simulink model "Control_Robot_using_Simulink"  (R2018b)
settings: Solver=FixedStepAuto  StartTime=0.0  StopTime=inf  FixedStep=0.01  RelTol=1e-3
undefined symbols (not defined in the file): Angular, Linear
libraries: robotlib x3, simulink x2
settings Model: Creator=chaitu  LastModifiedBy=chaitu

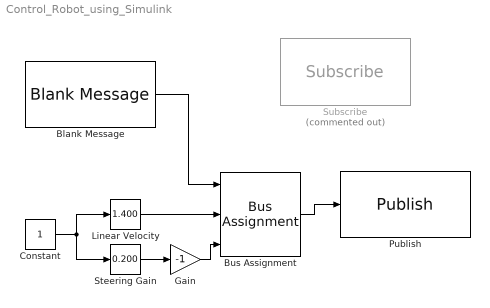
== system Control_Robot_using_Simulink ==
  Blank Message : robotlib/Blank Message  messageClass=Message  entityType=geometry_msgs/Twist  messageType=geometry_msgs/Twist  SampleTime=0.1
      settings: SourceProductBaseCode=RO
  Bus Assignment : BusAssignment  AssignedSignals=Linear.X,Angular.Z
  Constant : Constant
  Gain : Gain  Gain=-1
  Linear Velocity : simulink/Math Operations/Slider Gain  gain=1.400  low=0  high=2
  Publish : robotlib/Publish  topicSource=Select from ROS network  topic=/mobile_base/commands/velocity  messageType=geometry_msgs/Twist  messageQueueLength=1
      settings: SourceProductBaseCode=RO
  "Steering Gain " : simulink/Math Operations/Slider Gain  gain=0.200  low=-1  high=1
  Subscribe : robotlib/Subscribe  Commented=on  topicSource=Select from ROS network  topic=/odom  messageType=nav_msgs/Odometry  sampleTime=-1  messageQueueLength=1
      settings: SourceProductBaseCode=RO
  wires:
  Blank Message/1 -> Bus Assignment/1
  Bus Assignment/1 -> Publish/1
  Constant/1 -> Linear Velocity/1, "Steering Gain "/1
  Gain/1 -> Bus Assignment/3
  "Steering Gain "/1 -> Gain/1
  Linear Velocity/1 -> Bus Assignment/2
